simulink model "Validation"  (R2020b)
settings: Solver=VariableStepAuto  StartTime=0.0  StopTime=60  RelTol=1e-3
undefined symbols (not defined in the file or in its folder): InnerLoop
libraries: simulink x2
settings Model: Creator=Aurelien_Julien  LastModifiedBy=Aurelien_Julien

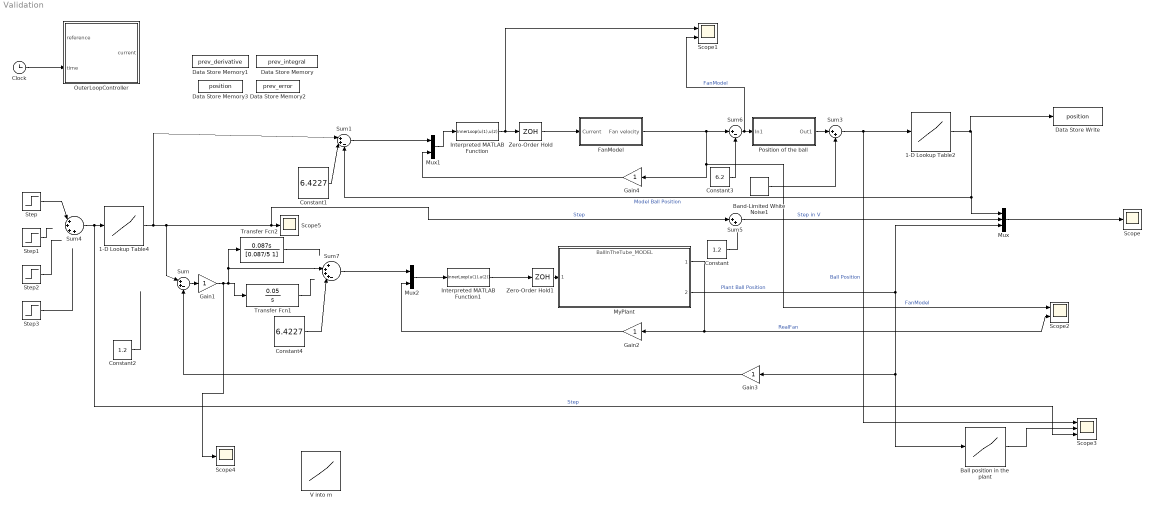
== system Validation ==
  1-D Lookup Table2 : Lookup_n-D  NumberOfTableDimensions=1  BreakpointsForDimension1=[0 15 60 97.5 117.5 125 127.5 132 135 138 142 148 152 160 167.5 180]/100  Table=[1.2 1.4 1.8 2.4 2.5 2.75 3.1 3.5 3.9 4.5 5.2 5.6 5.7 6.3 6.7 7.32]  InternalRulePriority=Speed  RndMeth=Simplest  InputSameDT=on
  1-D Lookup Table4 : Lookup_n-D  NumberOfTableDimensions=1  BreakpointsForDimension1=[0 15 60 97.5 117.5 125 127.5 132 135 138 142 148 152 160 167.5 180]/100  Table=[1.2 1.4 1.8 2.4 2.5 2.75 3.1 3.5 3.9 4.5 5.2 5.6 5.7 6.3 6.7 7.32]  InternalRulePriority=Speed  RndMeth=Simplest  InputSameDT=on
  Ball position in the plant : Lookup_n-D  NumberOfTableDimensions=1  BreakpointsForDimension1=[1.2 1.4 1.8 2.4 2.5 2.75 3.1 3.5 3.9 4.5 5.2 5.6 5.7 6.3 6.7 7.32]  Table=[0 15 60 97.5 117.5 125 127.5 132 135 138 142 148 152 160 167.5 180]/100  InternalRulePriority=Speed  RndMeth=Simplest  InputSameDT=on
  Band-Limited White Noise1 : simulink/Sources/Band-Limited White Noise  Cov=[0.0000001]  Ts=0.01  seed=[23341]
  Clock : Clock
  Constant : Constant  Value=1.2
  Constant1 : Constant  Value=6.4227
  Constant2 : Constant  Value=1.2
  Constant3 : Constant  Value=6.2
  Constant4 : Constant  Value=6.4227
  Data Store Memory : DataStoreMemory  DataStoreName=prev_integral  ReadBeforeWriteMsg=warning  WriteAfterWriteMsg=warning  WriteAfterReadMsg=warning  ShowAdditionalParam=off  OutDataTypeStr=double
  Data Store Memory1 : DataStoreMemory  DataStoreName=prev_derivative  ReadBeforeWriteMsg=warning  WriteAfterWriteMsg=warning  WriteAfterReadMsg=warning  ShowAdditionalParam=off  OutDataTypeStr=double
  Data Store Memory2 : DataStoreMemory  DataStoreName=prev_error  ReadBeforeWriteMsg=warning  WriteAfterWriteMsg=warning  WriteAfterReadMsg=warning  ShowAdditionalParam=off  OutDataTypeStr=double
  Data Store Memory3 : DataStoreMemory  DataStoreName=position  ReadBeforeWriteMsg=warning  WriteAfterWriteMsg=warning  WriteAfterReadMsg=warning  ShowAdditionalParam=off  OutDataTypeStr=double
  Data Store Write : DataStoreWrite  DataStoreName=position  SampleTime=0.01
  FanModel : Subsystem
  Gain{1..4} (4 alike) : Gain
  Interpreted MATLAB Function : MATLABFcn  MATLABFcn=InnerLoop(u(1),u(2))  OutputDimensions=1
  Interpreted MATLAB Function1 : MATLABFcn  MATLABFcn=InnerLoop(u(1),u(2))  OutputDimensions=1
  Mux : Mux  Inputs=3
  Mux1 : Mux  Inputs=2
  Mux2 : Mux  Inputs=2
  MyPlant : ModelReference  ModelNameDialog=BallInTheTube_MODEL  SimulationMode=Normal  ModelReferenceVersion=1.2
  OuterLoopController : MATLAB Function  TreatAsAtomicUnit=on  SystemSampleTime=0.01
  Position of the ball : Subsystem
  Scope : Scope
  Scope1 : Scope  NumInputPorts=2
  Scope2 : Scope  NumInputPorts=2
  Scope3 : Scope  NumInputPorts=3
  Scope4 : Scope
  Scope5 : Scope
  Step : Step  Time=20  After=0.5  SampleTime=0.01
  Step1 : Step  Time=30  After=0  SampleTime=0
  Step2 : Step  Time=45  After=-0.4  SampleTime=0
  Step3 : Step  Time=40  After=0.1  SampleTime=0
  Sum : Sum  Inputs=|++-
  Sum1 : Sum  Inputs=|++-
  Sum3 : Sum  Inputs=|++
  Sum4 : Sum  Inputs=|++++
  Sum5 : Sum  Inputs=|++
  Sum6 : Sum  Inputs=|+-
  Sum7 : Sum  Inputs=|++++-
  Transfer Fcn1 : TransferFcn  Numerator=[0.05]  Denominator=[1 0]
  Transfer Fcn2 : TransferFcn  Numerator=[0.087 0]  Denominator=[0.087/5 1]
  V into m : Lookup_n-D  NumberOfTableDimensions=1  BreakpointsForDimension1=[1.2 1.4 1.8 2.4 2.5 2.75 3.1 3.5 3.9 4.5 5.2 5.6 5.7 6.3 6.7 7.32]  Table=[0 15 60 97.5 117.5 125 127.5 132 135 138 142 148 152 160 167.5 180]/100  InternalRulePriority=Speed  RndMeth=Simplest  InputSameDT=on
  Zero-Order Hold : ZeroOrderHold  SampleTime=0.01
  Zero-Order Hold1 : ZeroOrderHold  SampleTime=0.01
  wires:
  Mux/1 -> Scope/1
  MyPlant/1 -> Gain2/1, Scope2/2  "RealFan"
  Gain3/1 -> Sum/3
  Zero-Order Hold/1 -> FanModel/1(Current)
  Interpreted MATLAB Function/1 -> Scope1/1, Zero-Order Hold/1
  Step/1 -> Sum4/1
  Step1/1 -> ?
  Gain4/1 -> Mux1/2
  Mux2/1 -> Interpreted MATLAB Function1/1
  Gain2/1 -> Mux2/2
  Position of the ball/1(Out1) -> Sum3/1
  Band-Limited White Noise1/1 -> Sum3/2
  Constant/1 -> ?
  Sum5/1 -> Mux/2  "Step in V"
  Mux1/1 -> Interpreted MATLAB Function/1
  Constant2/1 -> ?
  Zero-Order Hold1/1 -> MyPlant/1
  Ball position in the plant/1 -> Scope3/2
  Sum7/1 -> Mux2/1
  Constant4/1 -> Sum7/4
  Sum6/1 -> Scope1/2, Position of the ball/1(In1)  "FanModel"
  Step2/1 -> ?
  Constant3/1 -> Sum6/2
  FanModel/1(Fan velocity) -> Sum6/1, Scope2/1, Gain4/1  "FanModel"
  Sum1/1 -> Mux1/1
  Step3/1 -> ?
  Interpreted MATLAB Function1/1 -> Zero-Order Hold1/1
  Clock/1 -> OuterLoopController/2(time)
  Sum3/1 -> Scope3/1, 1-D Lookup Table2/1  "Ball Position"
  1-D Lookup Table2/1 -> Data Store Write/1, Sum1/3, Mux/1  "Model Ball Position"
  Sum/1 -> Gain1/1
  MyPlant/2 -> Ball position in the plant/1, Gain3/1, Mux/3  "Plant Ball Position"
  Constant1/1 -> Sum1/2
  Gain1/1 -> Scope4/1, Transfer Fcn1/1, Transfer Fcn2/1, Sum7/2
  Transfer Fcn1/1 -> ?
  Transfer Fcn2/1 -> ?
  Sum4/1 -> Scope3/3, 1-D Lookup Table4/1  "Step"
  1-D Lookup Table4/1 -> Sum1/1, Sum/1, Sum5/1, Scope5/1  "Step"

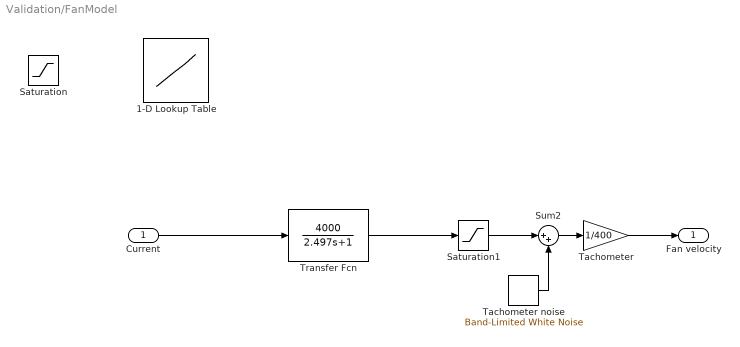
== system Validation/FanModel ==
  Current : Inport
  1-D Lookup Table : Lookup_n-D  NumberOfTableDimensions=1  BreakpointsForDimension1=[-4 -1 0 1 2 2.5 4]  Table=[-1450 -1300 0 1600 2800 3600 3800]  InternalRulePriority=Speed  RndMeth=Simplest  InputSameDT=on
  Saturation : Saturate  UpperLimit=7  LowerLimit=-7
  Saturation1 : Saturate  UpperLimit=9.6*400  LowerLimit=-3.6*400
  Sum2 : Sum  Inputs=|++
  Tachometer : Gain  Gain=1/400
  Tachometer noise : simulink/Sources/Band-Limited White Noise  Cov=[0.1]  Ts=0.01  seed=[23341]
  Transfer Fcn : TransferFcn  Numerator=[4000]  Denominator=[2.497 1]
  Fan velocity : Outport
  wires:
  Transfer Fcn/1 -> Saturation1/1
  Current/1 -> Transfer Fcn/1
  Tachometer/1 -> Fan velocity/1
  Tachometer noise/1 -> Sum2/2
  Saturation1/1 -> Sum2/1
  Sum2/1 -> Tachometer/1

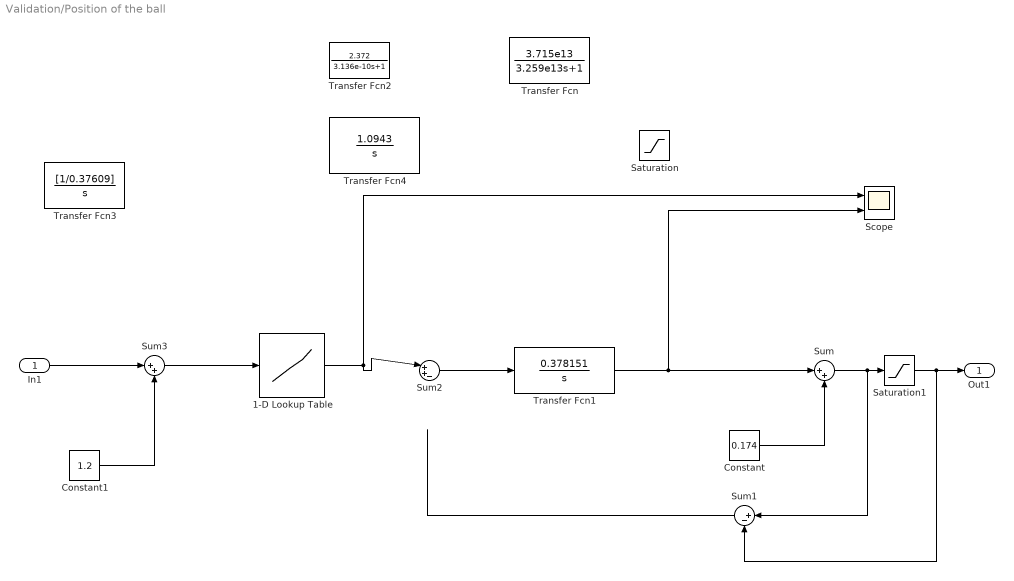
== system Validation/Position of the ball ==
  In1 : Inport
  1-D Lookup Table : Lookup_n-D  NumberOfTableDimensions=1  BreakpointsForDimension1=[1.2 1.4 1.8 2.4 2.5 2.75 3.1 3.5 3.9 4.5 5.2 5.6 5.7 6.3 6.7 7.32]  Table=[0 15 60 97.5 117.5 125 127.5 132 135 138 142 148 152 160 167.5 180]/100  InternalRulePriority=Speed  RndMeth=Simplest  InputSameDT=on
  Constant : Constant  Value=0.174
  Constant1 : Constant  Value=1.2
  Saturation : Saturate  UpperLimit=6.12  LowerLimit=0
  Saturation1 : Saturate  UpperLimit=1.8  LowerLimit=0
  Scope : Scope  NumInputPorts=2
  Sum : Sum  Inputs=|++
  Sum1 : Sum  Inputs=|+-
  Sum2 : Sum  Inputs=|++-
  Sum3 : Sum  Inputs=|++
  Transfer Fcn : TransferFcn  Numerator=[3.715e13]  Denominator=[3.259e13 1]
  Transfer Fcn1 : TransferFcn  Numerator=[0.378151]  Denominator=[1 0]
  Transfer Fcn2 : TransferFcn  Numerator=[2.372]  Denominator=[3.136e-10 1]
  Transfer Fcn3 : TransferFcn  Numerator=[1/0.37609]  Denominator=[1 0]
  Transfer Fcn4 : TransferFcn  Numerator=[1.0943]  Denominator=[1 0]
  Out1 : Outport
  wires:
  Constant/1 -> Sum/2
  Sum/1 -> Sum1/1, Saturation1/1
  Sum2/1 -> Transfer Fcn1/1
  Sum1/1 -> ?
  Constant1/1 -> Sum3/2
  Transfer Fcn1/1 -> Scope/2, Sum/1
  Saturation1/1 -> Sum1/2, Out1/1
  1-D Lookup Table/1 -> Sum2/1, Scope/1
  In1/1 -> Sum3/1
  Sum3/1 -> 1-D Lookup Table/1

== matlab function Validation/OuterLoopController ==
  data: reference input; current output; time input; prev_integral data_store_memory; prev_derivative data_store_memory; prev_error data_store_memory; position data_store_memory
function current = OuterLoopController(reference,time)
global prev_integral;
global prev_derivative;
global prev_error;
global position;

if(time == 0)
   prev_error = 0;
   prev_integral = 0;
   prev_derivative = 0;
end

Ki = 0.1;
Ts = 0.01;
Kd = 0.1;

if (position < 2.5)
    Kp = 5.0766;
else
    Kp = 0.70753;
end

error = reference - position;
integral = 0;
derivative = prev_derivative*0.5536+3.884*error-3.884*prev_error;
current = Kp*error + Kp*integral + Kp*derivative;

prev_integral = integral;
prev_derivative = derivative;
prev_error = error;

current = current + 6.4227;

if(abs(current)>10)
    current = 10*sign(current);
end

end
